simulink model "model_problem3"  (R2020a)
settings: Solver=VariableStepAuto  StartTime=0.0  StopTime=100.0  RelTol=1e-3
settings Model: Creator=Prateek  LastModifiedBy=Prateek

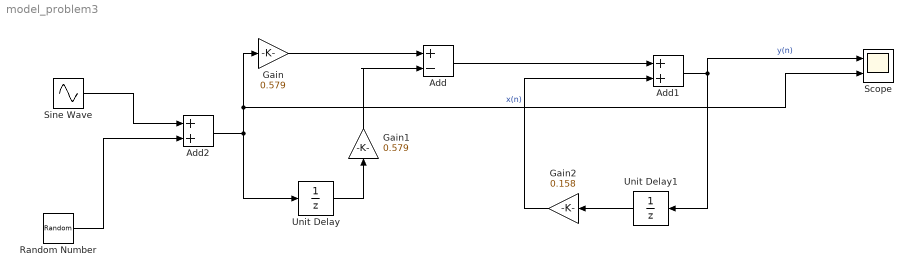
== system model_problem3 ==
  Add : Sum  Inputs=+-
  Add1 : Sum
  Add2 : Sum
  Gain : Gain  Gain=0.579
  Gain1 : Gain  Gain=0.579
  Gain2 : Gain  Gain=0.158
  Random Number : RandomNumber  SampleTime=0.001
  Scope : Scope  NumInputPorts=2
  Sine Wave : Sin  SampleTime=0
  Unit Delay : UnitDelay  SampleTime=-1  HasFrameUpgradeWarning=on
  Unit Delay1 : UnitDelay  SampleTime=-1  HasFrameUpgradeWarning=on
  wires:
  Gain/1 -> Add/1
  Unit Delay/1 -> Gain1/1
  Gain1/1 -> Add/2
  Add2/1 -> Gain/1, Scope/2, Unit Delay/1  "x(n)"
  Add/1 -> Add1/1
  Add1/1 -> Scope/1, Unit Delay1/1  "y(n)"
  Unit Delay1/1 -> Gain2/1
  Gain2/1 -> Add1/2
  Sine Wave/1 -> Add2/1
  Random Number/1 -> Add2/2
